simulink model "PWM_Motor_Driver_Circuit"  (R2014b)
settings: Solver=ode45  StartTime=0.0  StopTime=.3  MaxStep=.0001  RelTol=1e-3

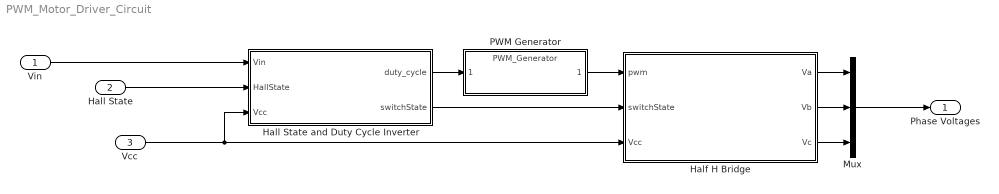
== system PWM_Motor_Driver_Circuit ==
  Vin : Inport  OutDataTypeStr=double  PortDimensions=1  SampleTime=0
  Hall State : Inport  Port=2
  Vcc : Inport  Port=3  OutDataTypeStr=double  PortDimensions=1  SampleTime=[0, 0]
  Half H Bridge : MATLAB Function  TreatAsAtomicUnit=on
  Hall State and Duty Cycle Inverter : MATLAB Function  TreatAsAtomicUnit=on
  Mux : Mux  Inputs=3
  PWM Generator : ModelReference  ModelNameDialog=PWM_Generator  SimulationMode=Normal  ModelReferenceVersion=1.162  CopyOfModelName=PWM_Generator  DefaultDataLogging=on
  Phase Voltages : Outport  OutDataTypeStr=double  PortDimensions=3  SampleTime=0
  wires:
  Vcc/1 -> Hall State and Duty Cycle Inverter/3(Vcc), Half H Bridge/3(Vcc)
  PWM Generator/1 -> Half H Bridge/1(pwm)
  Hall State and Duty Cycle Inverter/2(switchState) -> Half H Bridge/2(switchState)
  Vin/1 -> Hall State and Duty Cycle Inverter/1(Vin)
  Hall State and Duty Cycle Inverter/1(duty_cycle) -> PWM Generator/1
  Half H Bridge/3(Vc) -> Mux/3
  Half H Bridge/2(Vb) -> Mux/2
  Half H Bridge/1(Va) -> Mux/1
  Mux/1 -> Phase Voltages/1
  Hall State/1 -> Hall State and Duty Cycle Inverter/2(HallState)

== matlab function PWM_Motor_Driver_Circuit/Half H Bridge ==
function [Va, Vb, Vc] = HalfHBridge(pwm, switchState, Vcc)
    if isequal(switchState, [1, 0, 0])
        Va = pwm*Vcc;
        Vb = 0;
        Vc = pwm*Vcc/2;
    elseif isequal(switchState, [1, 1, 0])
        Va = pwm*Vcc;
        Vb = pwm*Vcc/2;
        Vc = 0;
    elseif isequal(switchState, [0, 1, 0])
        Va = pwm*Vcc/2
        Vb = pwm*Vcc;
        Vc = 0;
    elseif isequal(switchState, [0, 1, 1])
        Va = 0;
        Vb = pwm*Vcc;
        Vc = pwm*Vcc/2;
   elseif isequal(switchState, [0, 0, 1])
        Va = 0;
        Vb = pwm*Vcc/2;
        Vc = pwm*Vcc;
    elseif isequal(switchState, [1, 0, 1])
        Va = pwm*Vcc/2;
        Vb = 0;
        Vc = pwm*Vcc;
    else
        Va = 0;
        Vb = 0;
        Vc = 0;
end

== matlab function PWM_Motor_Driver_Circuit/Hall State and Duty Cycle Inverter ==
function [duty_cycle, switchState] = hallStateInv(Vin, HallState, Vcc)
duty_cycle = Vin/Vcc;
if (duty_cycle < 0)
    duty_cycle = abs(duty_cycle);
    switchState = -1*HallState + [1, 1, 1]; %%Ghetto way of invertering Hallstate                                     %%if the duty cycle is negative
else
    switchState = HallState;
end
